simulink model "linear_actuator_le"  (R2020a)
settings: Solver=ode45  StartTime=0.0  StopTime=simlength  MaxStep=1e-4  RelTol=1e-4
undefined symbols (not defined in the file): A, Aled, B, Bled, C, Cle, E, Ked, Lled, Tc, Ts
settings Model: Creator=dabagnara  LastModifiedBy=dbagn
settings DataIOCC: ReturnWorkspaceOutputs=off

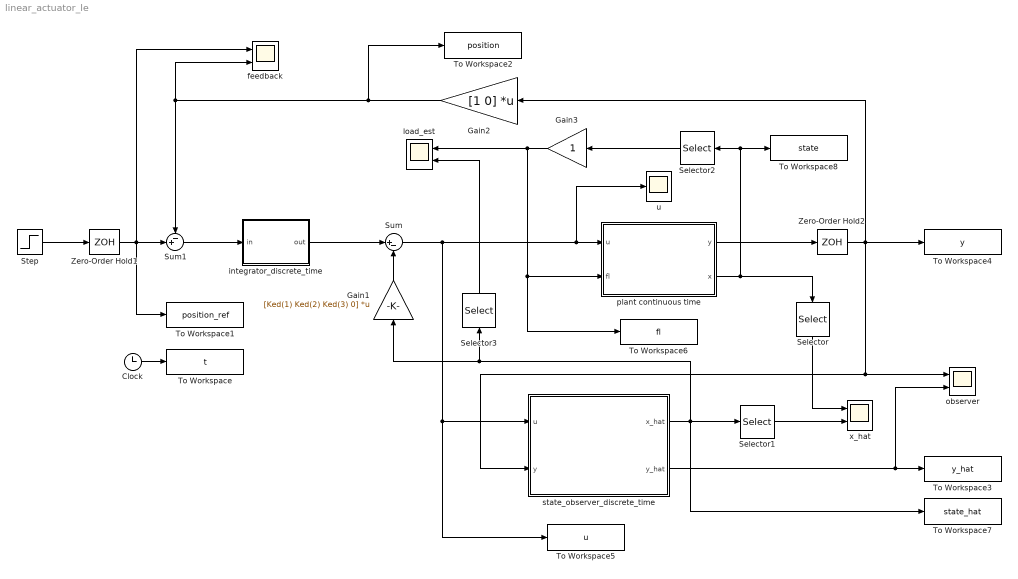
== system linear_actuator_le ==
  Clock : Clock
  Gain1 : Gain  Gain=[Ked(1) Ked(2) Ked(3) 0]  Multiplication=Matrix(K*u)
  Gain2 : Gain  Gain=[1 0]  Multiplication=Matrix(K*u)
  Gain3 : Gain
  Selector : Selector  InputPortWidth=3  IndexOptions=Index vector (dialog)  Indices=2  OutputSizes=1
  Selector1 : Selector  InputPortWidth=4  IndexOptions=Index vector (dialog)  Indices=2  OutputSizes=1
  Selector2 : Selector  InputPortWidth=3  IndexOptions=Index vector (dialog)  Indices=2  OutputSizes=1
  Selector3 : Selector  InputPortWidth=4  IndexOptions=Index vector (dialog)  Indices=4  OutputSizes=1
  Step : Step  Time=0.1  SampleTime=0
  Sum : Sum  Inputs=|+-
  Sum1 : Sum  Inputs=-+|
  To Workspace : ToWorkspace  VariableName=t  SampleTime=Tc
      settings: MaxDataPoints=Nc
  To Workspace1 : ToWorkspace  VariableName=position_ref  SampleTime=Tc
      settings: MaxDataPoints=Nc
  To Workspace2 : ToWorkspace  VariableName=position  SampleTime=Tc
      settings: MaxDataPoints=Nc
  To Workspace3 : ToWorkspace  VariableName=y_hat  SampleTime=Tc
      settings: MaxDataPoints=Nc
  To Workspace4 : ToWorkspace  VariableName=y  SampleTime=Tc
      settings: MaxDataPoints=Nc
  To Workspace5 : ToWorkspace  VariableName=u  SampleTime=Tc
      settings: MaxDataPoints=Nc
  To Workspace6 : ToWorkspace  VariableName=fl  SampleTime=Tc
      settings: MaxDataPoints=Nc
  To Workspace7 : ToWorkspace  VariableName=state_hat  SampleTime=Tc
      settings: MaxDataPoints=Nc
  To Workspace8 : ToWorkspace  VariableName=state  SampleTime=Tc
      settings: MaxDataPoints=Nc
  Zero-Order Hold1 : ZeroOrderHold  SampleTime=Ts
  Zero-Order Hold2 : ZeroOrderHold  SampleTime=Ts
  feedback : Scope  NumInputPorts=2
  integrator_discrete_time : Subsystem
  load_est : Scope  NumInputPorts=2
  observer : Scope  NumInputPorts=2
  plant continuous time : Subsystem
  state_observer_discrete_time : Subsystem
  u : Scope
  x_hat : Scope  NumInputPorts=2
  wires:
  Sum1/1 -> integrator_discrete_time/1(in)
  Zero-Order Hold2/1 -> state_observer_discrete_time/2(y), observer/1, To Workspace4/1, Gain2/1
  Sum/1 -> u/1, plant continuous time/1(u), To Workspace5/1, state_observer_discrete_time/1(u)
  Clock/1 -> To Workspace/1
  Gain2/1 -> Sum1/1, feedback/2, To Workspace2/1
  Zero-Order Hold1/1 -> To Workspace1/1, feedback/1, Sum1/2
  state_observer_discrete_time/2(y_hat) -> To Workspace3/1, observer/2
  state_observer_discrete_time/1(x_hat) -> Selector1/1, To Workspace7/1, Selector3/1, Gain1/1
  Step/1 -> Zero-Order Hold1/1
  integrator_discrete_time/1(out) -> Sum/1
  Gain1/1 -> Sum/2
  Gain3/1 -> plant continuous time/2(fl), To Workspace6/1, load_est/1
  plant continuous time/2(x) -> To Workspace8/1, Selector2/1, Selector/1
  Selector/1 -> x_hat/1
  Selector1/1 -> x_hat/2
  Selector2/1 -> Gain3/1
  plant continuous time/1(y) -> Zero-Order Hold2/1
  Selector3/1 -> load_est/2

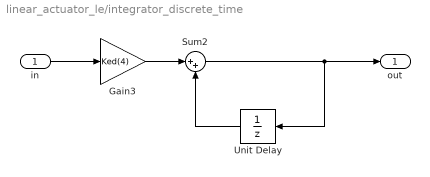
== system linear_actuator_le/integrator_discrete_time ==
  in : Inport
  Gain3 : Gain  Gain=Ked(4)
  Sum2 : Sum  Inputs=|++
  Unit Delay : UnitDelay  SampleTime=Ts  HasFrameUpgradeWarning=on
  out : Outport
  wires:
  Sum2/1 -> out/1, Unit Delay/1
  in/1 -> Gain3/1
  Gain3/1 -> Sum2/1
  Unit Delay/1 -> Sum2/2

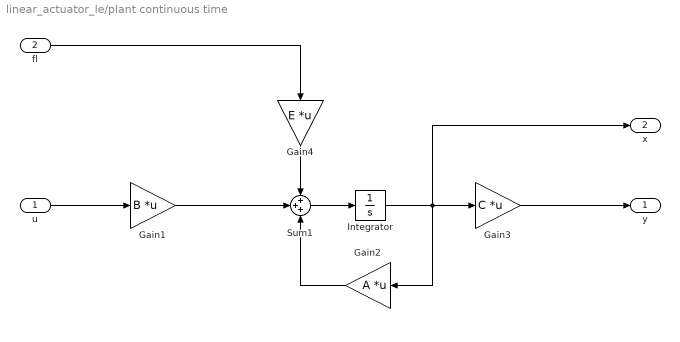
== system linear_actuator_le/plant continuous time ==
  u : Inport
  fl : Inport  Port=2
  Gain1 : Gain  Gain=B  Multiplication=Matrix(K*u)
  Gain2 : Gain  Gain=A  Multiplication=Matrix(K*u)
  Gain3 : Gain  Gain=C  Multiplication=Matrix(K*u)
  Gain4 : Gain  Gain=E  Multiplication=Matrix(K*u)
  Integrator : Integrator
  Sum1 : Sum  Inputs=+++
  y : Outport
  x : Outport  Port=2
  wires:
  Sum1/1 -> Integrator/1
  u/1 -> Gain1/1
  Integrator/1 -> x/1, Gain2/1, Gain3/1
  Gain3/1 -> y/1
  Gain2/1 -> Sum1/3
  Gain1/1 -> Sum1/2
  Gain4/1 -> Sum1/1
  fl/1 -> Gain4/1

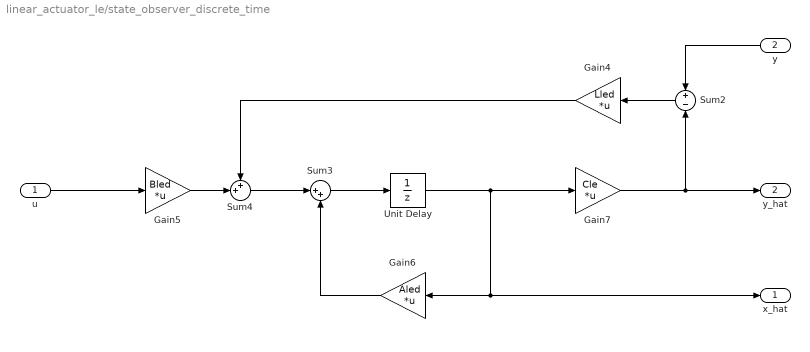
== system linear_actuator_le/state_observer_discrete_time ==
  u : Inport
  y : Inport  Port=2
  Gain4 : Gain  Gain=Lled  Multiplication=Matrix(K*u)
  Gain5 : Gain  Gain=Bled  Multiplication=Matrix(K*u)
  Gain6 : Gain  Gain=Aled  Multiplication=Matrix(K*u)
  Gain7 : Gain  Gain=Cle  Multiplication=Matrix(K*u)
  Sum2 : Sum  Inputs=+-
  Sum3 : Sum  Inputs=|++
  Sum4 : Sum  Inputs=++|
  Unit Delay : UnitDelay  SampleTime=Ts  HasFrameUpgradeWarning=on
  x_hat : Outport
  y_hat : Outport  Port=2
  wires:
  Gain7/1 -> y_hat/1, Sum2/2
  Unit Delay/1 -> Gain7/1, Gain6/1, x_hat/1
  Sum3/1 -> Unit Delay/1
  Gain4/1 -> Sum4/1
  y/1 -> Sum2/1
  Gain5/1 -> Sum4/2
  Sum2/1 -> Gain4/1
  Gain6/1 -> Sum3/2
  Sum4/1 -> Sum3/1
  u/1 -> Gain5/1
